simulink model "day2"  (R2024a)
settings: Solver=VariableStepAuto  StartTime=0.0  StopTime=10.0  RelTol=1e-3
libraries: simulink_extras x24, commrandsrc3 x1
settings Model: Creator=tusha  LastModifiedBy=tusha

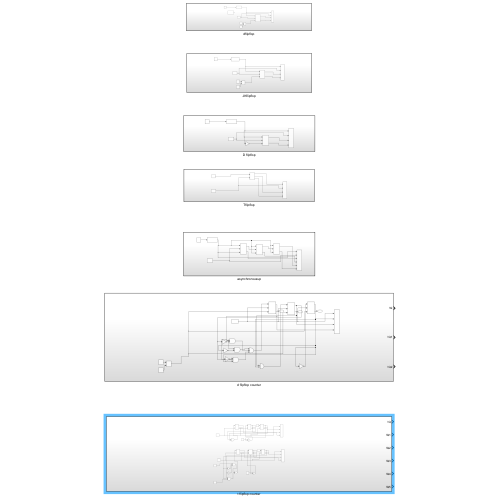
[thumbnail: Simulink's stored preview of the top-level diagram]
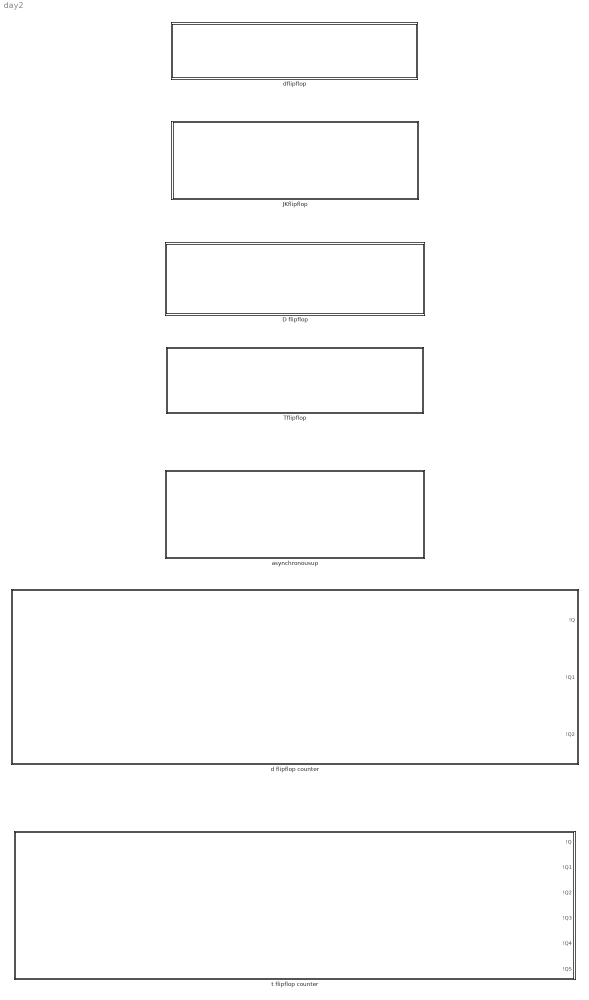
== system day2 ==
  D flipflop : Subsystem
  JKflipflop : Subsystem
  Tflipflop : Subsystem
  asynchronousup : Subsystem
  d flipflop counter : Subsystem
  dflipflop : Subsystem
  t flipflop counter : Subsystem

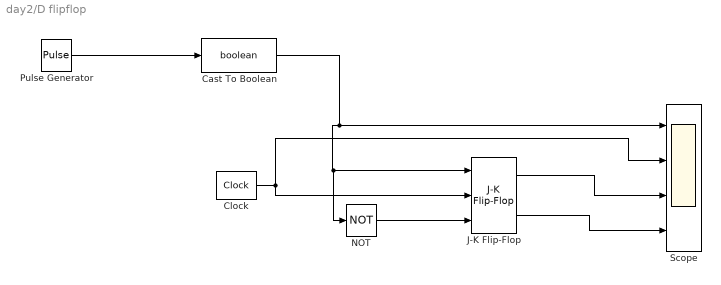
== system day2/D flipflop ==
  Cast To Boolean : DataTypeConversion  OutDataTypeStr=boolean  SaturateOnIntegerOverflow=off  RndMeth=Floor
  Clock : simulink_extras/Flip Flops/Clock  period=0.5
  J-K Flip-Flop : simulink_extras/Flip Flops/J-K Flip-Flop  initial_condition=0
  NOT : Logic  Operator=NOT  IconShape=distinctive  AllPortsSameDT=off  OutDataTypeStr=boolean
  Pulse Generator : DiscretePulseGenerator  PulseType=Time based  PulseWidth=50
  Scope : Scope  NumInputPorts=4
  wires:
  Pulse Generator/1 -> Cast To Boolean/1
  J-K Flip-Flop/2 -> Scope/4
  Clock/1 -> J-K Flip-Flop/2, Scope/2
  Cast To Boolean/1 -> NOT/1, J-K Flip-Flop/1, Scope/1
  NOT/1 -> J-K Flip-Flop/3
  J-K Flip-Flop/1 -> Scope/3

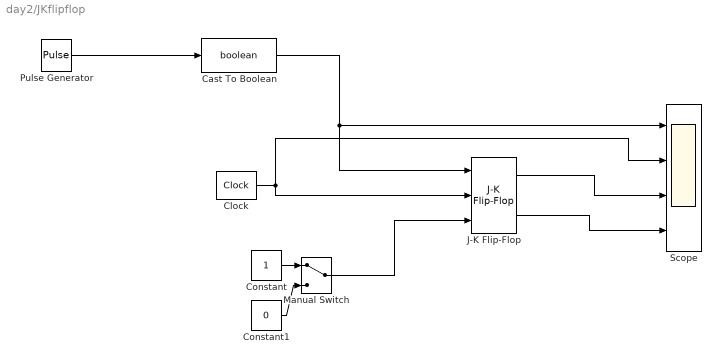
== system day2/JKflipflop ==
  Cast To Boolean : DataTypeConversion  OutDataTypeStr=boolean  SaturateOnIntegerOverflow=off  RndMeth=Floor
  Clock : simulink_extras/Flip Flops/Clock  period=0.5
  Constant : Constant  OutDataTypeStr=boolean
  Constant1 : Constant  Value=0  OutDataTypeStr=boolean
  J-K Flip-Flop : simulink_extras/Flip Flops/J-K Flip-Flop  initial_condition=0
  Manual Switch : ManualSwitch
  Pulse Generator : DiscretePulseGenerator  PulseType=Time based  PulseWidth=50
  Scope : Scope  NumInputPorts=4
  wires:
  Manual Switch/1 -> J-K Flip-Flop/3
  Cast To Boolean/1 -> J-K Flip-Flop/1, Scope/1
  Constant1/1 -> Manual Switch/2
  Pulse Generator/1 -> Cast To Boolean/1
  Clock/1 -> J-K Flip-Flop/2, Scope/2
  Constant/1 -> Manual Switch/1
  J-K Flip-Flop/1 -> Scope/3
  J-K Flip-Flop/2 -> Scope/4

== system day2/Tflipflop ==
  Clock : simulink_extras/Flip Flops/Clock  period=0.5
  Pulse Generator : DiscretePulseGenerator  PulseType=Time based  PulseWidth=50
  Scope : Scope  NumInputPorts=4
  Subsystem : Subsystem
  wires:
  Clock/1 -> Subsystem/2(CLK), Scope/2
  Pulse Generator/1 -> Subsystem/1(In1)
  Subsystem/1(J) -> Scope/1
  Subsystem/2(Q) -> Scope/3
  Subsystem/3(!Q) -> Scope/4

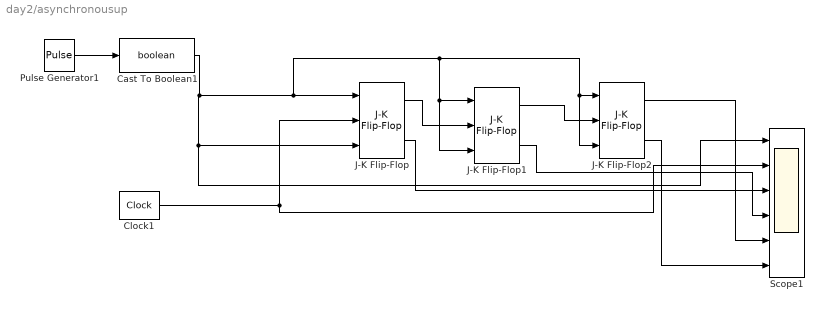
== system day2/asynchronousup ==
  Cast To Boolean1 : DataTypeConversion  OutDataTypeStr=boolean  SaturateOnIntegerOverflow=off  RndMeth=Floor
  Clock1 : simulink_extras/Flip Flops/Clock  period=2
  J-K Flip-Flop : simulink_extras/Flip Flops/J-K Flip-Flop  initial_condition=0
  J-K Flip-Flop1 : simulink_extras/Flip Flops/J-K Flip-Flop  initial_condition=0
  J-K Flip-Flop2 : simulink_extras/Flip Flops/J-K Flip-Flop  initial_condition=0
  Pulse Generator1 : DiscretePulseGenerator  PulseType=Time based  PulseWidth=50
  Scope1 : Scope  NumInputPorts=6
  wires:
  Pulse Generator1/1 -> Cast To Boolean1/1
  Cast To Boolean1/1 -> Scope1/1, J-K Flip-Flop/3, J-K Flip-Flop2/3, J-K Flip-Flop2/1, J-K Flip-Flop1/3, J-K Flip-Flop1/1, J-K Flip-Flop/1
  J-K Flip-Flop1/1 -> J-K Flip-Flop2/2
  Clock1/1 -> J-K Flip-Flop/2, Scope1/2
  J-K Flip-Flop1/2 -> Scope1/4
  J-K Flip-Flop2/2 -> Scope1/6
  J-K Flip-Flop/1 -> J-K Flip-Flop1/2
  J-K Flip-Flop/2 -> Scope1/3
  J-K Flip-Flop2/1 -> Scope1/5

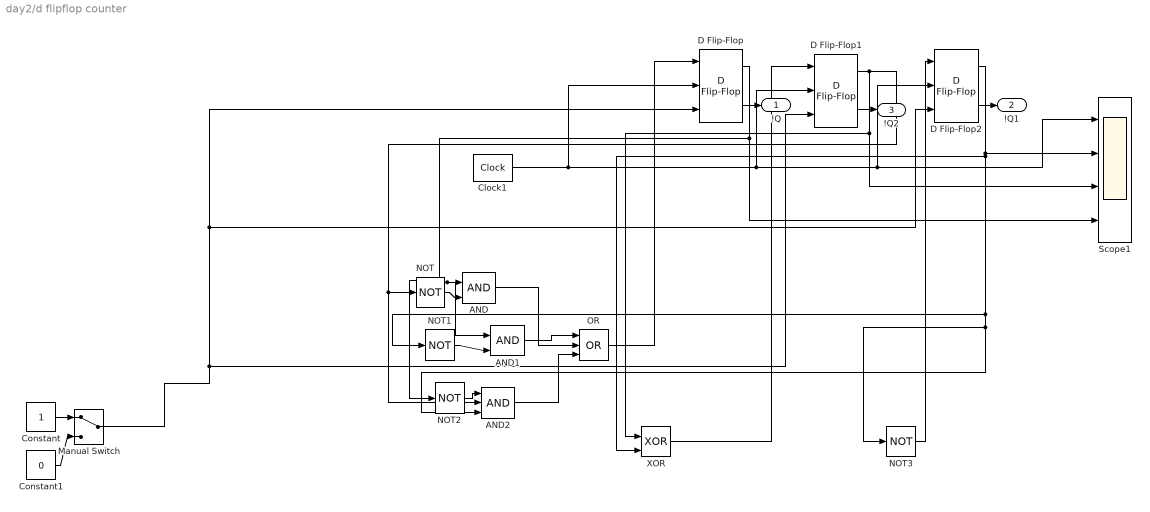
== system day2/d flipflop counter ==
  AND : Logic  IconShape=distinctive  AllPortsSameDT=off  OutDataTypeStr=boolean
  AND1 : Logic  IconShape=distinctive  AllPortsSameDT=off  OutDataTypeStr=boolean
  AND2 : Logic  Inputs=3  IconShape=distinctive  AllPortsSameDT=off  OutDataTypeStr=boolean
  Clock1 : simulink_extras/Flip Flops/Clock  period=0.5
  Constant : Constant  OutDataTypeStr=boolean
  Constant1 : Constant  Value=0  OutDataTypeStr=boolean
  D Flip-Flop : simulink_extras/Flip Flops/D Flip-Flop
  D Flip-Flop1 : simulink_extras/Flip Flops/D Flip-Flop
  D Flip-Flop2 : simulink_extras/Flip Flops/D Flip-Flop
  Manual Switch : ManualSwitch
  NOT{,1..3} (4 alike) : Logic  Operator=NOT  IconShape=distinctive  AllPortsSameDT=off  OutDataTypeStr=boolean
  OR : Logic  Operator=OR  Inputs=3  IconShape=distinctive  AllPortsSameDT=off  OutDataTypeStr=boolean
  Scope1 : Scope  NumInputPorts=4
  XOR : Logic  Operator=XOR  IconShape=distinctive  AllPortsSameDT=off  OutDataTypeStr=boolean
  !Q : Outport
  !Q1 : Outport  Port=2
  !Q2 : Outport  Port=3
  wires:
  D Flip-Flop/2 -> !Q/1
  D Flip-Flop/1 -> Scope1/4, NOT2/1, AND1/1, AND/1
  Manual Switch/1 -> D Flip-Flop2/3, D Flip-Flop/3, D Flip-Flop1/3
  Clock1/1 -> D Flip-Flop/2, D Flip-Flop1/2, Scope1/1, D Flip-Flop2/2
  NOT2/1 -> AND2/1
  AND1/1 -> OR/1
  AND2/1 -> OR/3
  OR/1 -> D Flip-Flop/1
  D Flip-Flop2/1 -> Scope1/2, NOT3/1, AND2/3, NOT1/1, XOR/2
  D Flip-Flop1/1 -> Scope1/3, XOR/1, AND2/2, NOT/1
  NOT3/1 -> D Flip-Flop2/1
  Constant/1 -> Manual Switch/1
  AND/1 -> OR/2
  XOR/1 -> D Flip-Flop1/1
  NOT/1 -> AND/2
  D Flip-Flop2/2 -> !Q1/1
  D Flip-Flop1/2 -> !Q2/1
  NOT1/1 -> AND1/2
  Constant1/1 -> Manual Switch/2

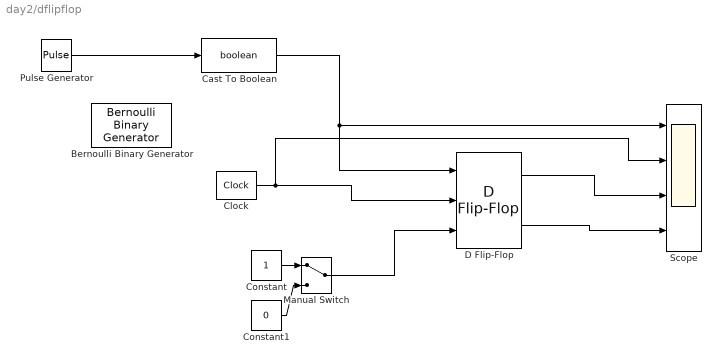
== system day2/dflipflop ==
  Bernoulli Binary Generator : commrandsrc3/Bernoulli Binary Generator  ProbabilityOfZero=0.5  SeedSource=Auto  Seed=0  SampleTime=1  SamplesPerFrame=1  OutputDataType=boolean  SimulateUsing=Interpreted execution
  Cast To Boolean : DataTypeConversion  OutDataTypeStr=boolean  SaturateOnIntegerOverflow=off  RndMeth=Floor
  Clock : simulink_extras/Flip Flops/Clock  period=0.5
  Constant : Constant  OutDataTypeStr=boolean
  Constant1 : Constant  Value=0  OutDataTypeStr=boolean
  D Flip-Flop : simulink_extras/Flip Flops/D Flip-Flop
  Manual Switch : ManualSwitch
  Pulse Generator : DiscretePulseGenerator  PulseType=Time based  PulseWidth=50
  Scope : Scope  NumInputPorts=4
  wires:
  Manual Switch/1 -> D Flip-Flop/3
  D Flip-Flop/2 -> Scope/4
  Constant/1 -> Manual Switch/1
  Clock/1 -> Scope/2, D Flip-Flop/2
  Constant1/1 -> Manual Switch/2
  D Flip-Flop/1 -> Scope/3
  Cast To Boolean/1 -> D Flip-Flop/1, Scope/1
  Pulse Generator/1 -> Cast To Boolean/1

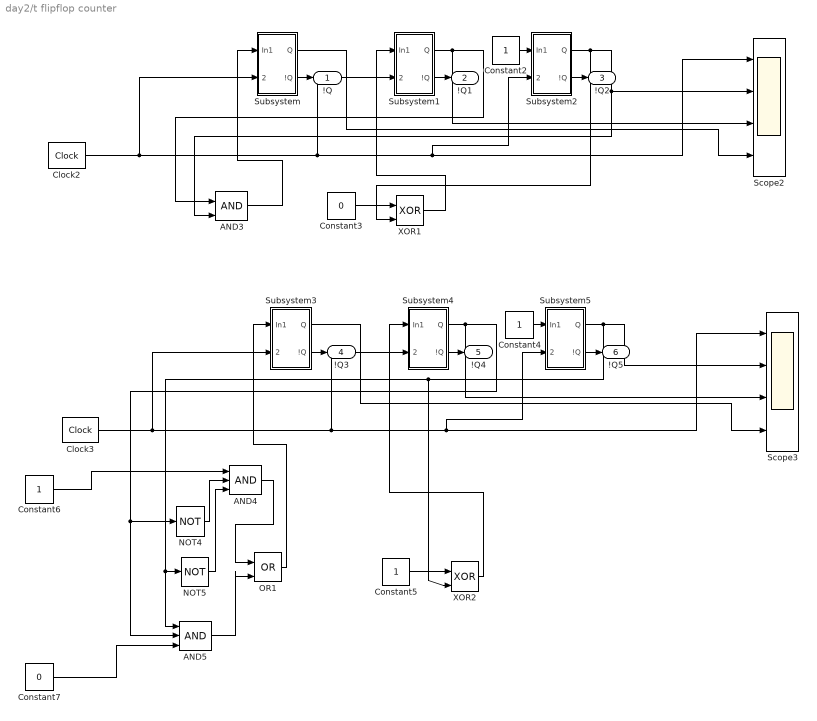
== system day2/t flipflop counter ==
  AND3 : Logic  IconShape=distinctive  AllPortsSameDT=off  OutDataTypeStr=boolean
  AND4 : Logic  Inputs=3  IconShape=distinctive  AllPortsSameDT=off  OutDataTypeStr=boolean
  AND5 : Logic  Inputs=3  IconShape=distinctive  AllPortsSameDT=off  OutDataTypeStr=boolean
  Clock2 : simulink_extras/Flip Flops/Clock  period=0.5
  Clock3 : simulink_extras/Flip Flops/Clock  period=0.5
  Constant{2,4..6} (4 alike) : Constant
  Constant3 : Constant  Value=0
  Constant7 : Constant  Value=0
  NOT4 : Logic  Operator=NOT  IconShape=distinctive  AllPortsSameDT=off  OutDataTypeStr=boolean
  NOT5 : Logic  Operator=NOT  IconShape=distinctive  AllPortsSameDT=off  OutDataTypeStr=boolean
  OR1 : Logic  Operator=OR  IconShape=distinctive  AllPortsSameDT=off  OutDataTypeStr=boolean
  Scope2 : Scope  NumInputPorts=4
  Scope3 : Scope  NumInputPorts=4
  Subsystem : Subsystem
  Subsystem1 : Subsystem
  Subsystem2 : Subsystem
  Subsystem3 : Subsystem
  Subsystem4 : Subsystem
  Subsystem5 : Subsystem
  XOR1 : Logic  Operator=XOR  IconShape=distinctive  AllPortsSameDT=off  OutDataTypeStr=boolean
  XOR2 : Logic  Operator=XOR  IconShape=distinctive  AllPortsSameDT=off  OutDataTypeStr=boolean
  !Q : Outport
  !Q1 : Outport  Port=2
  !Q2 : Outport  Port=3
  !Q3 : Outport  Port=4
  !Q4 : Outport  Port=5
  !Q5 : Outport  Port=6
  wires:
  Subsystem1/1(Q) -> Scope2/3, AND3/1
  Constant4/1 -> Subsystem5/1(In1)
  Constant5/1 -> XOR2/1
  XOR1/1 -> Subsystem1/1(In1)
  NOT5/1 -> AND4/3
  Constant6/1 -> AND4/1
  Subsystem2/1(Q) -> XOR1/2, AND3/2, Scope2/2
  Subsystem3/1(Q) -> Scope3/4
  Subsystem5/1(Q) -> AND5/1, NOT5/1, XOR2/2, Scope3/2
  Clock3/1 -> Subsystem3/2(CLK), Subsystem4/2(CLK), Scope3/1, Subsystem5/2(CLK)
  Subsystem4/1(Q) -> AND5/2, NOT4/1, Scope3/3
  XOR2/1 -> Subsystem4/1(In1)
  Clock2/1 -> Subsystem/2(CLK), Subsystem1/2(CLK), Scope2/1, Subsystem2/2(CLK)
  Subsystem/2(!Q) -> !Q/1
  Subsystem4/2(!Q) -> !Q4/1
  Constant2/1 -> Subsystem2/1(In1)
  Subsystem5/2(!Q) -> !Q5/1
  Subsystem/1(Q) -> Scope2/4
  Subsystem2/2(!Q) -> !Q2/1
  AND3/1 -> Subsystem/1(In1)
  OR1/1 -> Subsystem3/1(In1)
  AND5/1 -> OR1/2
  Constant3/1 -> XOR1/1
  Constant7/1 -> AND5/3
  NOT4/1 -> AND4/2
  AND4/1 -> OR1/1
  Subsystem3/2(!Q) -> !Q3/1
  Subsystem1/2(!Q) -> !Q1/1

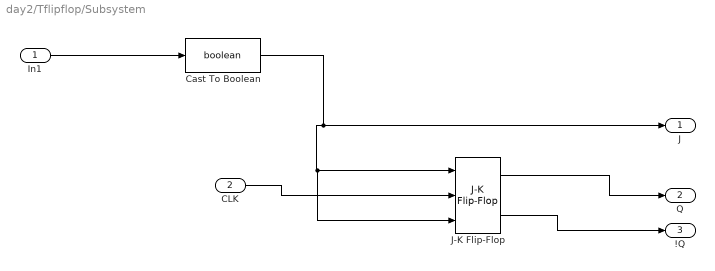
== system day2/Tflipflop/Subsystem ==
  In1 : Inport
  CLK : Inport  Port=2
  Cast To Boolean : DataTypeConversion  OutDataTypeStr=boolean  SaturateOnIntegerOverflow=off  RndMeth=Floor
  J-K Flip-Flop : simulink_extras/Flip Flops/J-K Flip-Flop  initial_condition=0
  J : Outport
  Q : Outport  Port=2
  !Q : Outport  Port=3
  wires:
  J-K Flip-Flop/2 -> !Q/1
  CLK/1 -> J-K Flip-Flop/2
  J-K Flip-Flop/1 -> Q/1
  Cast To Boolean/1 -> J/1, J-K Flip-Flop/3, J-K Flip-Flop/1
  In1/1 -> Cast To Boolean/1

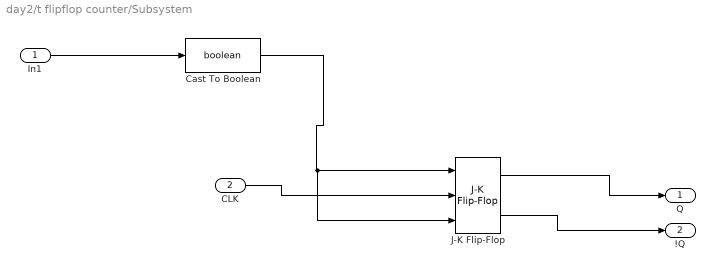
== system day2/t flipflop counter/Subsystem ==
  In1 : Inport
  CLK : Inport  Port=2
  Cast To Boolean : DataTypeConversion  OutDataTypeStr=boolean  SaturateOnIntegerOverflow=off  RndMeth=Floor
  J-K Flip-Flop : simulink_extras/Flip Flops/J-K Flip-Flop  initial_condition=0
  Q : Outport
  !Q : Outport  Port=2
  wires:
  J-K Flip-Flop/2 -> !Q/1
  CLK/1 -> J-K Flip-Flop/2
  J-K Flip-Flop/1 -> Q/1
  Cast To Boolean/1 -> J-K Flip-Flop/3, J-K Flip-Flop/1
  In1/1 -> Cast To Boolean/1

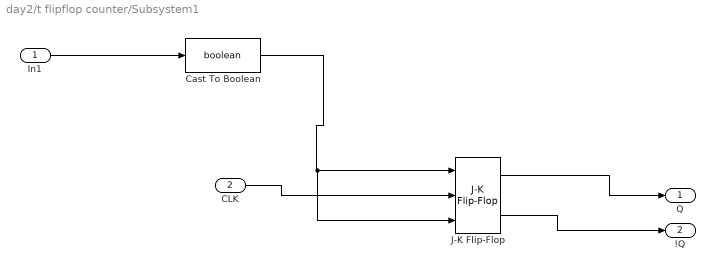
== system day2/t flipflop counter/Subsystem1 ==
  In1 : Inport
  CLK : Inport  Port=2
  Cast To Boolean : DataTypeConversion  OutDataTypeStr=boolean  SaturateOnIntegerOverflow=off  RndMeth=Floor
  J-K Flip-Flop : simulink_extras/Flip Flops/J-K Flip-Flop  initial_condition=0
  Q : Outport
  !Q : Outport  Port=2
  wires:
  J-K Flip-Flop/2 -> !Q/1
  CLK/1 -> J-K Flip-Flop/2
  J-K Flip-Flop/1 -> Q/1
  Cast To Boolean/1 -> J-K Flip-Flop/3, J-K Flip-Flop/1
  In1/1 -> Cast To Boolean/1

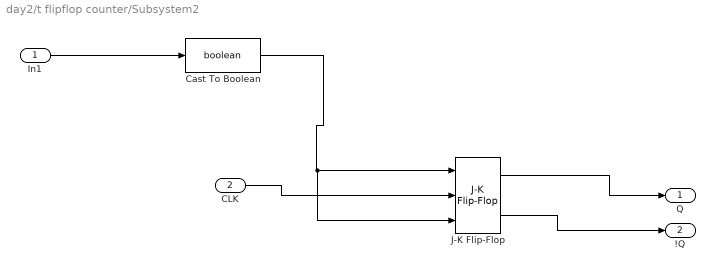
== system day2/t flipflop counter/Subsystem2 ==
  In1 : Inport
  CLK : Inport  Port=2
  Cast To Boolean : DataTypeConversion  OutDataTypeStr=boolean  SaturateOnIntegerOverflow=off  RndMeth=Floor
  J-K Flip-Flop : simulink_extras/Flip Flops/J-K Flip-Flop  initial_condition=0
  Q : Outport
  !Q : Outport  Port=2
  wires:
  J-K Flip-Flop/2 -> !Q/1
  CLK/1 -> J-K Flip-Flop/2
  J-K Flip-Flop/1 -> Q/1
  Cast To Boolean/1 -> J-K Flip-Flop/3, J-K Flip-Flop/1
  In1/1 -> Cast To Boolean/1

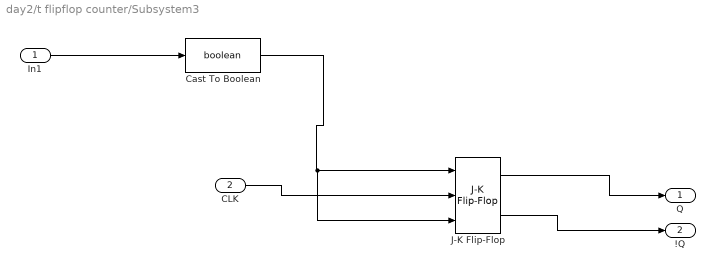
== system day2/t flipflop counter/Subsystem3 ==
  In1 : Inport
  CLK : Inport  Port=2
  Cast To Boolean : DataTypeConversion  OutDataTypeStr=boolean  SaturateOnIntegerOverflow=off  RndMeth=Floor
  J-K Flip-Flop : simulink_extras/Flip Flops/J-K Flip-Flop  initial_condition=0
  Q : Outport
  !Q : Outport  Port=2
  wires:
  J-K Flip-Flop/2 -> !Q/1
  CLK/1 -> J-K Flip-Flop/2
  J-K Flip-Flop/1 -> Q/1
  Cast To Boolean/1 -> J-K Flip-Flop/3, J-K Flip-Flop/1
  In1/1 -> Cast To Boolean/1

== system day2/t flipflop counter/Subsystem4 ==
  In1 : Inport
  CLK : Inport  Port=2
  Cast To Boolean : DataTypeConversion  OutDataTypeStr=boolean  SaturateOnIntegerOverflow=off  RndMeth=Floor
  J-K Flip-Flop : simulink_extras/Flip Flops/J-K Flip-Flop  initial_condition=0
  Q : Outport
  !Q : Outport  Port=2
  wires:
  J-K Flip-Flop/2 -> !Q/1
  CLK/1 -> J-K Flip-Flop/2
  J-K Flip-Flop/1 -> Q/1
  Cast To Boolean/1 -> J-K Flip-Flop/3, J-K Flip-Flop/1
  In1/1 -> Cast To Boolean/1

== system day2/t flipflop counter/Subsystem5 ==
  In1 : Inport
  CLK : Inport  Port=2
  Cast To Boolean : DataTypeConversion  OutDataTypeStr=boolean  SaturateOnIntegerOverflow=off  RndMeth=Floor
  J-K Flip-Flop : simulink_extras/Flip Flops/J-K Flip-Flop  initial_condition=0
  Q : Outport
  !Q : Outport  Port=2
  wires:
  J-K Flip-Flop/2 -> !Q/1
  CLK/1 -> J-K Flip-Flop/2
  J-K Flip-Flop/1 -> Q/1
  Cast To Boolean/1 -> J-K Flip-Flop/3, J-K Flip-Flop/1
  In1/1 -> Cast To Boolean/1
